simulink model "DashboardIntegration"  (R2021b)
settings: Solver=FixedStepAuto  StartTime=0.0  StopTime=10.0  FixedStep=0.2  RelTol=1e-3
libraries: simulink x1
settings Model: Creator=ajfem  LastModifiedBy=ajfem

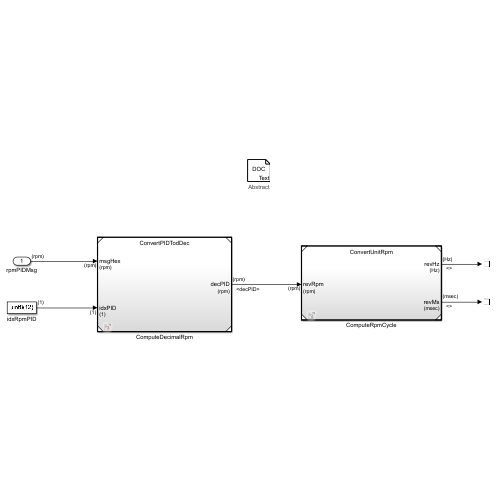
[thumbnail: Simulink's stored preview of the top-level diagram]
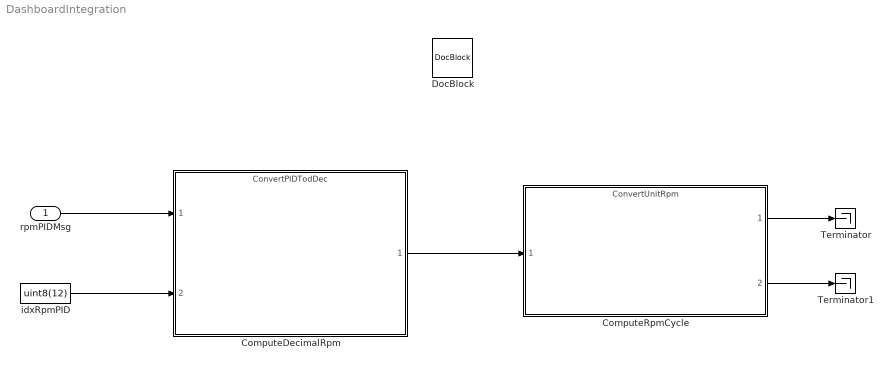
== system DashboardIntegration ==
  rpmPIDMsg : Inport  OutDataTypeStr=double  Unit=rpm  PortDimensions=1
  ComputeDecimalRpm : ModelReference  ModelNameDialog=ConvertPIDTodDec.slx  SimulationMode=Normal  ModelReferenceVersion=1.19
  ComputeRpmCycle : ModelReference  ModelNameDialog=ConvertUnitRpm.slx  SimulationMode=Normal  ModelReferenceVersion=1.11
  DocBlock : simulink/Model-Wide Utilities/DocBlock  ECoderFlag=Abstract  DocumentType=Text
      content=|
      | Integration for full model functionality.
      settings: AttributesFormatString=%<ECoderFlag>
  Terminator : Terminator
  Terminator1 : Terminator
  idxRpmPID : Constant  Value=uint8(12)
  wires:
  rpmPIDMsg/1 -> ComputeDecimalRpm/1
  idxRpmPID/1 -> ComputeDecimalRpm/2
  ComputeDecimalRpm/1 -> ComputeRpmCycle/1
  ComputeRpmCycle/1 -> Terminator/1
  ComputeRpmCycle/2 -> Terminator1/1
